simulink model "algorithm"  (R2026a)
settings: Solver=FixedStepDiscrete  FixedStep=foc.Ts
PreLoadFcn:
  | if exist('init', 'file') ~= 2,   pDir = fileparts(fileparts(which(bdroot)));   if isempty(pDir), pDir = pwd; end;   addpath(fullfile(pDir, 'scripts'));   addpath(fullfile(pDir, 'models'));   addpath(pDir); end; init;
InitFcn:
  | if exist('init', 'file') ~= 2,   pDir = fileparts(fileparts(which(bdroot)));   if isempty(pDir), pDir = pwd; end;   addpath(fullfile(pDir, 'scripts'));   addpath(fullfile(pDir, 'models'));   addpath(pDir); end; init;
undefined symbols (not defined in the file): calibration_modulation, calibration_request, control_enable_request, control_fault_reset, control_mode_request, current_offset_counts, DiscIntNeverNeededParam, foc, has_stored_resolver_offset, open_loop_electrical_hz, open_loop_modulation, pmsm, resolver_angle_offset, sensor, torque_ref_nm
libraries: mcbeeMathTransformLib x3, slpidlib x3, mcbcontrolslib x3, simulink x2, mcbpositiondecoderlib x1
(part 1 of 2)
settings Model: Creator=niklasprobst  LastModifiedBy=probst
settings OptimizationCC: DefaultUnderspecifiedDataType=single
settings DebuggingCC: ParameterDowncastMsg=none  ParameterPrecisionLossMsg=none  BusObjectLabelMismatch=error
settings RTWCC: SystemTargetFile=ert.tlc  GenCodeOnly=on  Description=Embedded Coder
settings ERTTargetCC: SupportAbsoluteTime=off  SupportNonFinite=off

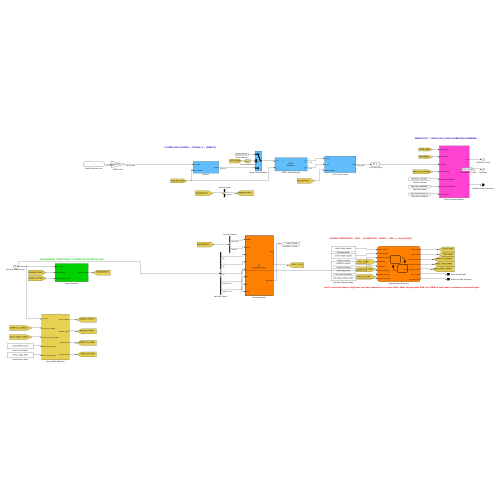
[thumbnail: Simulink's stored preview of the top-level diagram]
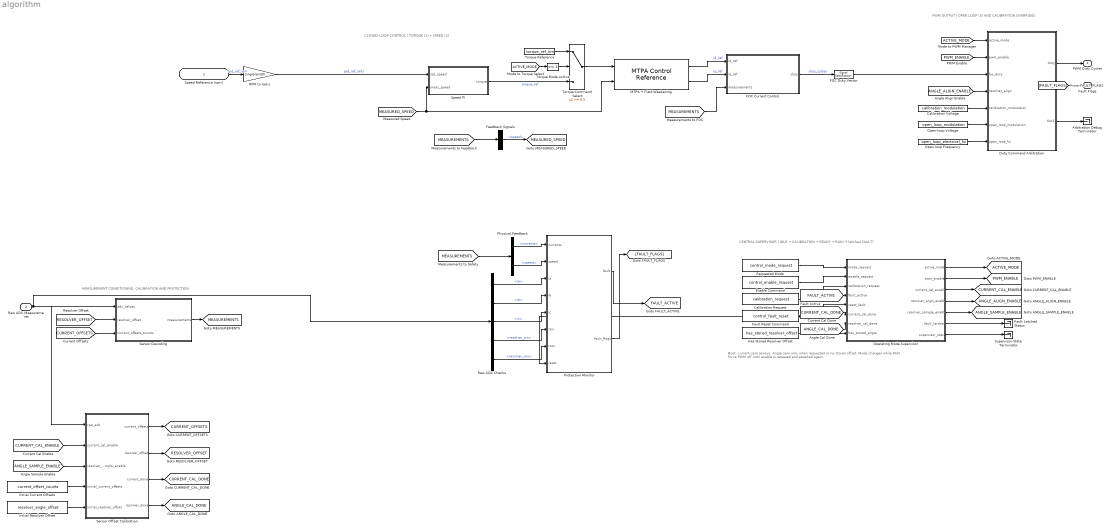
== system algorithm ==
  note: CLOSED-LOOP CONTROL | TORQUE (1) • SPEED (2)
  note: PWM OUTPUT | OPEN LOOP (3) AND CALIBRATION OVERRIDES
  note: MEASUREMENT CONDITIONING, CALIBRATION AND PROTECTION
  note: CENTRAL SUPERVISOR | IDLE → CALIBRATION → READY → RUN (+ latched FAULT)
  note: Boot: current-zero always. Angle-zero only when requested or no stored offset. Mode changes while RUN force PWM off until enable is released and asserted again.
  Speed Reference (rpm) : Inport  OutDataTypeStr=single
  Raw ADC Measurements : Inport  Port=2  OutDataTypeStr=Bus: adc_values
  Arbitration Debug Terminator : Terminator
      settings: Tag=algorithm_clean_routing
  Calibration Request : Constant  Value=calibration_request  OutDataTypeStr=uint8
  Calibration Voltage : Constant  Value=calibration_modulation  OutDataTypeStr=single
  Duty Command Arbitration : Subsystem
  Enable Command : Constant  Value=control_enable_request  OutDataTypeStr=boolean
  FOC Current Control : Subsystem
  FOC Duty Vector : SignalSpecification  Dimensions=3
  Fault Latched Status : Terminator
  Fault Reset Command : Constant  Value=control_fault_reset  OutDataTypeStr=boolean
  Feedback Signals : BusSelector  OutputSignals=speed
  Has Stored Resolver Offset : Constant  Value=has_stored_resolver_offset  OutDataTypeStr=boolean
  Initial Current Offsets : Constant  Value=current_offset_counts  OutDataTypeStr=single
  Initial Resolver Offset : Constant  Value=resolver_angle_offset  OutDataTypeStr=single
  MTPA + Field Weakening : mcbcontrolslib/MTPA Control Reference  VariantSelect=Interior PMSM  polePairs=pmsm.P  Rs=pmsm.Rs  Ld=pmsm.Ld  Lq=pmsm.Lq  FluxPM=pmsm.fl  ilimit=pmsm.I_rated  Vdc_input_select=Specify via dialog  V_dc=pmsm.V_rated  Units=SI Units  N_base=pmsm.N_base  I_base=pmsm.I_rated  T_base=1  V_base=pmsm.V_rated/sqrt(3)  N_base_disp=pmsm.N_base  MTPAiterator=on  iterCount=10
  Open-loop Frequency : Constant  Value=open_loop_electrical_hz  OutDataTypeStr=single
  Open-loop Voltage : Constant  Value=open_loop_modulation  OutDataTypeStr=single
  Operating Mode Supervisor : Stateflow chart  TreatAsAtomicUnit=on
  Physical Feedback : BusSelector  OutputSignals=currents,speed
  Protection Monitor : MATLAB Function  TreatAsAtomicUnit=on
  RPM to rad-s : Gain  Gain=single(pi/30)  OutDataTypeStr=single
  Raw ADC Checks : BusSelector  OutputSignals=ia,ib,ic,resolver_sin,resolver_cos
  Requested Mode : Constant  Value=control_mode_request  OutDataTypeStr=uint8
  Sensor Decoding : Subsystem  Description=|
      | EVADC TO PHYSICAL SENSOR MEASUREMENT CONDITIONING
      | =================================================
      | 1. WHAT IT DOES:
      | Hardware abstraction interface that transforms raw 12-bit integer counts from the
      | Infineon AURIX TC387 EVADC into single-precision physical SI measurements packed into
      | the 'algo_measurement' bus.
      | 
      | 2. INTERFACE SIGNALS:
      | - Input:  'adc_values' bus (uint16 channels: ia, ib, ic, resolver_sin, resolver_cos)
      | - Output: 'measurements' bus (algo_measurement):
      |     * currents [A]    : 3-phase stator currents (Phase A, B, C)
      |     * MtrPos   [rad]  : Mechanical rotor angle in [0, 2*pi)
      |     * speed    [rad/s]: Filtered mechanical rotor speed
      | 
      | 3. INTERNAL SUBMODULES:
      |   1) Current measurement: Signed offset removal & scaling (0..4095 counts -> -120..+120 A).
      |   2) Position measurement: Center removal, normalization, atan2, and [0, 2*pi) wrapping.
      |   3) Speed from position: Differentiator with circular 2*pi unwrapping & 150 Hz LPF.
      | 
      | 4. WHY IT IS NEEDED:
      | Decouples microcontroller register hardware formats from core FOC algorithms, ensuring
      | pure single-precision floating-point execution, determinism, and seamless code generation.
      | Execution rate: Ts = 50 us (20 kHz).
  Sensor Offset Calibration : Subsystem
  Speed PI : Subsystem
  Supervisor State Terminator : Terminator
  Torque Command Select : Switch  Threshold=0.5  SaturateOnIntegerOverflow=off  InputSameDT=off
  Torque Mode Active : simulink/Logic and Bit Operations/Compare To Constant  relop===  const=1  OutDataTypeStr=boolean
  Torque Reference : Constant  Value=torque_ref_nm  OutDataTypeStr=single
  PWM Duty Cycles : Outport  OutDataTypeStr=single
  Fault Flags : Outport  Port=2  OutDataTypeStr=uint32
  tag scope: ACTIVE_MODE=global, ANGLE_ALIGN_ENABLE=global, ANGLE_CAL_DONE=global, ANGLE_SAMPLE_ENABLE=global, CURRENT_CAL_DONE=global, CURRENT_CAL_ENABLE=global, CURRENT_OFFSETS=global, FAULT_ACTIVE=global, MEASURED_SPEED=global, MEASUREMENTS=global, PWM_ENABLE=global, RESOLVER_OFFSET=global
  wires:
  Speed Reference (rpm)/1 -> RPM to rad-s/1  "spd_ref_rpm"
  RPM to rad-s/1 -> Speed PI/1(set_speed)  "spd_ref_rads"
  [MEASURED_SPEED] -> Speed PI/2(meas_speed), MTPA + Field Weakening/2
  Torque Reference/1 -> Torque Command Select/1
  [ACTIVE_MODE] -> Torque Mode Active/1
  Torque Mode Active/1 -> Torque Command Select/2
  Speed PI/1(torque) -> Torque Command Select/3  "torque_ref"
  Torque Command Select/1 -> MTPA + Field Weakening/1
  MTPA + Field Weakening/1 -> FOC Current Control/1(id_ref)  "id_ref"
  MTPA + Field Weakening/2 -> FOC Current Control/2(iq_ref)  "iq_ref"
  [MEASUREMENTS] -> FOC Current Control/3(measurements)
  FOC Current Control/1(duty) -> FOC Duty Vector/1  "duty_cycles"
  FOC Duty Vector/1 -> Duty Command Arbitration/3(foc_duty)
  [ACTIVE_MODE] -> Duty Command Arbitration/1(active_mode)
  [PWM_ENABLE] -> Duty Command Arbitration/2(pwm_enable)
  [ANGLE_ALIGN_ENABLE] -> Duty Command Arbitration/4(resolver_align)
  Calibration Voltage/1 -> Duty Command Arbitration/5(calibration_modulation)
  Open-loop Voltage/1 -> Duty Command Arbitration/6(open_loop_modulation)
  Open-loop Frequency/1 -> Duty Command Arbitration/7(open_loop_hz)
  Duty Command Arbitration/1(duty) -> PWM Duty Cycles/1
  Duty Command Arbitration/2(Out1) -> Arbitration Debug Terminator/1
  Sensor Decoding/1(measurements) -> [MEASUREMENTS]
  [RESOLVER_OFFSET] -> Sensor Decoding/2(resolver_offset)
  [CURRENT_OFFSETS] -> Sensor Decoding/3(current_offsets_counts)
  [MEASUREMENTS] -> Feedback Signals/1
  Feedback Signals/1 -> [MEASURED_SPEED]  "<speed>"
  [MEASUREMENTS] -> Physical Feedback/1
  Physical Feedback/1 -> Protection Monitor/1(currents)  "<currents>"
  Physical Feedback/2 -> Protection Monitor/2(speed)  "<speed>"
  Raw ADC Checks/1 -> Protection Monitor/3(ia)  "<ia>"
  Raw ADC Checks/2 -> Protection Monitor/4(ib)  "<ib>"
  Raw ADC Checks/3 -> Protection Monitor/5(ic)  "<ic>"
  Raw ADC Checks/4 -> Protection Monitor/6(rsin)  "<resolver_sin>"
  Raw ADC Checks/5 -> Protection Monitor/7(rcos)  "<resolver_cos>"
  Protection Monitor/1(fault) -> [FAULT_ACTIVE]
  [CURRENT_CAL_ENABLE] -> Sensor Offset Calibration/2(current_cal_enable)
  [ANGLE_SAMPLE_ENABLE] -> Sensor Offset Calibration/3(resolver_sample_enable)
  Initial Current Offsets/1 -> Sensor Offset Calibration/4(initial_current_offsets)
  Initial Resolver Offset/1 -> Sensor Offset Calibration/5(initial_resolver_offset)
  Sensor Offset Calibration/1(current_offsets) -> [CURRENT_OFFSETS]
  Sensor Offset Calibration/2(resolver_offset) -> [RESOLVER_OFFSET]
  Sensor Offset Calibration/3(current_done) -> [CURRENT_CAL_DONE]
  Sensor Offset Calibration/4(resolver_done) -> [ANGLE_CAL_DONE]
  Requested Mode/1 -> Operating Mode Supervisor/1(mode_request)
  Enable Command/1 -> Operating Mode Supervisor/2(enable_request)
  Calibration Request/1 -> Operating Mode Supervisor/3(calibration_request)
  [FAULT_ACTIVE] -> Operating Mode Supervisor/4(fault_active)
  Fault Reset Command/1 -> Operating Mode Supervisor/5(reset_fault), Protection Monitor/8(reset)
  [CURRENT_CAL_DONE] -> Operating Mode Supervisor/6(current_cal_done)
  [ANGLE_CAL_DONE] -> Operating Mode Supervisor/7(resolver_cal_done)
  Has Stored Resolver Offset/1 -> Operating Mode Supervisor/8(has_stored_angle)
  Operating Mode Supervisor/1(active_mode) -> [ACTIVE_MODE]
  Operating Mode Supervisor/2(pwm_enable) -> [PWM_ENABLE]
  Operating Mode Supervisor/3(current_cal_enable) -> [CURRENT_CAL_ENABLE]
  Operating Mode Supervisor/4(resolver_align_enable) -> [ANGLE_ALIGN_ENABLE]
  Operating Mode Supervisor/5(resolver_sample_enable) -> [ANGLE_SAMPLE_ENABLE]
  Operating Mode Supervisor/6(fault_latched) -> Fault Latched Status/1
  Operating Mode Supervisor/7(supervisor_state) -> Supervisor State Terminator/1
  Raw ADC Measurements/1 -> Sensor Decoding/1(adc_values), Sensor Offset Calibration/1(raw_adc), Raw ADC Checks/1
  Protection Monitor/2(fault_flags) -> [FAULT_FLAGS]
  [FAULT_FLAGS] -> Fault Flags/1

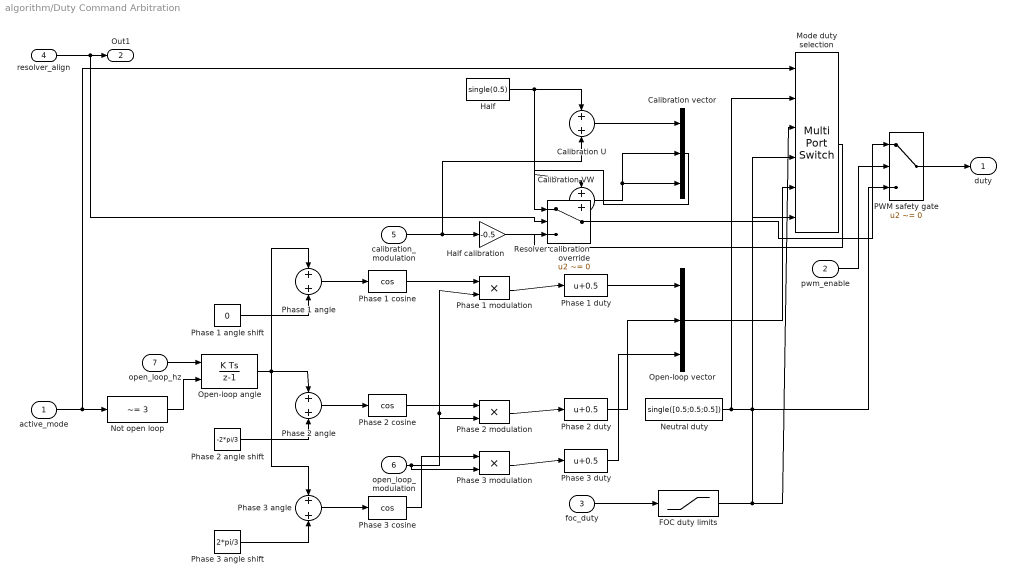
== system algorithm/Duty Command Arbitration ==
  active_mode : Inport
  pwm_enable : Inport  Port=2
  foc_duty : Inport  Port=3
  resolver_align : Inport  Port=4
  calibration_modulation : Inport  Port=5
  open_loop_modulation : Inport  Port=6
  open_loop_hz : Inport  Port=7
  Calibration U : Sum
  Calibration VW : Sum
  Calibration vector : Mux  Inputs=3
  FOC duty limits : Saturate  UpperLimit=0.98  LowerLimit=0.02
  Half : Constant  Value=single(0.5)
  Half calibration : Gain  Gain=-0.5
  Mode duty selection : MultiPortSwitch  DataPortOrder=Zero-based contiguous  Inputs=5  zeroidx=on  SaturateOnIntegerOverflow=off  InputSameDT=off
  Neutral duty : Constant  Value=single([0.5;0.5;0.5])
  Not open loop : simulink/Logic and Bit Operations/Compare To Constant  relop=~=  const=3  OutDataTypeStr=boolean
  Open-loop angle : DiscreteIntegrator  gainval=2*pi  ExternalReset=rising  SampleTime=foc.Ts  LimitOutput=on  UpperSaturationLimit=2*pi  LowerSaturationLimit=0  ICPrevOutput=DiscIntNeverNeededParam  ICPrevScaledInput=DiscIntNeverNeededParam
  Open-loop vector : Mux  Inputs=3
  PWM safety gate : Switch  Criteria=u2 ~= 0  Threshold=0.5  SaturateOnIntegerOverflow=off  InputSameDT=off
  Phase 1 angle : Sum
  Phase 1 angle shift : Constant  Value=0
  Phase 1 cosine : Trigonometry  Operator=cos
  Phase 1 duty : Bias  Bias=0.5  SaturateOnIntegerOverflow=off
  Phase 1 modulation : Product
  Phase 2 angle : Sum
  Phase 2 angle shift : Constant  Value=-2*pi/3
  Phase 2 cosine : Trigonometry  Operator=cos
  Phase 2 duty : Bias  Bias=0.5  SaturateOnIntegerOverflow=off
  Phase 2 modulation : Product
  Phase 3 angle : Sum
  Phase 3 angle shift : Constant  Value=2*pi/3
  Phase 3 cosine : Trigonometry  Operator=cos
  Phase 3 duty : Bias  Bias=0.5  SaturateOnIntegerOverflow=off
  Phase 3 modulation : Product
  Resolver calibration override : Switch  Criteria=u2 ~= 0  SaturateOnIntegerOverflow=off  InputSameDT=off
  duty : Outport
  Out1 : Outport  Port=2
  wires:
  PWM safety gate/1 -> duty/1
  pwm_enable/1 -> PWM safety gate/2
  Neutral duty/1 -> PWM safety gate/3, Mode duty selection/6, Mode duty selection/2
  foc_duty/1 -> FOC duty limits/1
  Phase 3 duty/1 -> Open-loop vector/3
  Phase 2 duty/1 -> Open-loop vector/2
  Phase 1 duty/1 -> Open-loop vector/1
  Half/1 -> Calibration U/1, Calibration VW/1
  Calibration U/1 -> Calibration vector/1
  Calibration VW/1 -> Calibration vector/3, Calibration vector/2
  Phase 3 cosine/1 -> Phase 3 modulation/1
  Phase 3 modulation/1 -> Phase 3 duty/1
  open_loop_modulation/1 -> Phase 2 modulation/2, Phase 1 modulation/2, Phase 3 modulation/2
  Half calibration/1 -> Calibration VW/2
  Phase 2 cosine/1 -> Phase 2 modulation/1
  Phase 1 cosine/1 -> Phase 1 modulation/1
  Phase 1 modulation/1 -> Phase 1 duty/1
  calibration_modulation/1 -> Half calibration/1, Calibration U/2
  Phase 2 modulation/1 -> Phase 2 duty/1
  Phase 3 angle/1 -> Phase 3 cosine/1
  Phase 3 angle shift/1 -> Phase 3 angle/2
  Open-loop angle/1 -> Phase 3 angle/1, Phase 1 angle/1, Phase 2 angle/1
  Phase 1 angle shift/1 -> Phase 1 angle/2
  Not open loop/1 -> Open-loop angle/2
  Phase 1 angle/1 -> Phase 1 cosine/1
  open_loop_hz/1 -> Open-loop angle/1
  active_mode/1 -> Not open loop/1, Mode duty selection/1
  resolver_align/1 -> Out1/1, Resolver calibration override/2
  Phase 2 angle shift/1 -> Phase 2 angle/2
  Phase 2 angle/1 -> Phase 2 cosine/1
  FOC duty limits/1 -> Mode duty selection/3, Mode duty selection/4
  Open-loop vector/1 -> Mode duty selection/5
  Calibration vector/1 -> Resolver calibration override/1
  Mode duty selection/1 -> Resolver calibration override/3
  Resolver calibration override/1 -> PWM safety gate/1

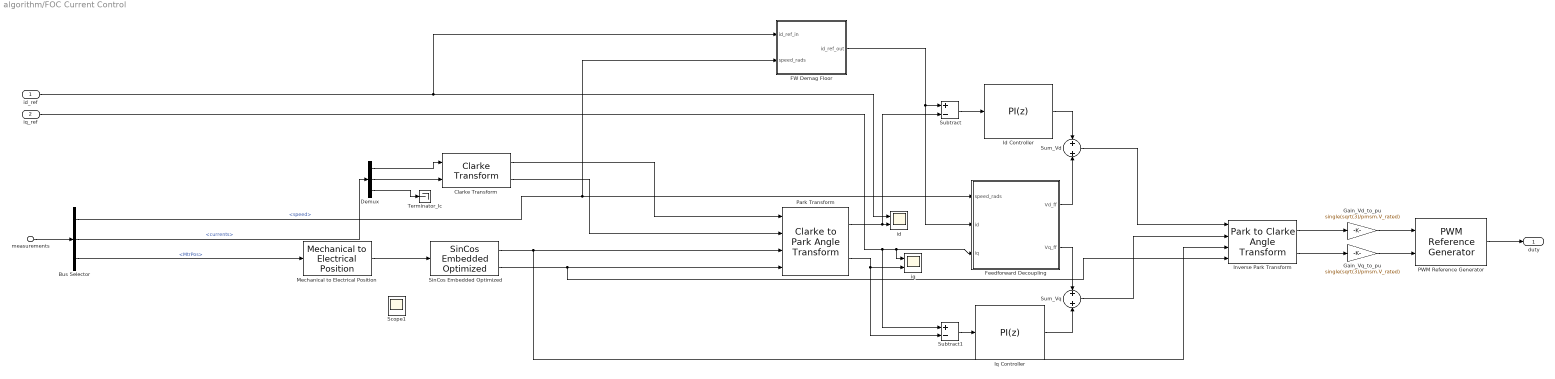
== system algorithm/FOC Current Control ==
  id_ref : Inport
  iq_ref : Inport  Port=2
  measurements : Inport  Port=3  OutDataTypeStr=Bus: algo_measurement
  Bus Selector : BusSelector  OutputSignals=speed,currents,MtrPos
  Clarke Transform : mcbeeMathTransformLib/Clarke Transform  VariantControl=Variant2  PowerInvariant=off  UseWithEmbedded=on  PhaseInput=Two inputs
      settings: LibrarySourceBlock=mcblib/Controls/Math Transforms/Clarke Transform
  Demux : Demux  Outputs=[1 1 1]
  FW Demag Floor : Subsystem  Description=|
      | FIELD WEAKENING DEMAGNETIZATION FLOOR (PHYSICAL VOLTAGE ENVELOPE)
      | =================================================================
      | 1. WHAT IT DOES:
      | Computes the maximum permissible stator flux linkage for the current rotor speed
      | given the inverter voltage headroom, calculates the minimum negative d-axis
      | demagnetization current required to stay within that flux limit, and enforces this
      | floor on id_ref.
      | 
      | 2. MATHEMATICAL FORMULAS:
      |   omega_e      = P * |omega_m|
      |   omega_e_safe = max(omega_e, 100 rad/s)          [Zero-speed division guard]
      |   V_max        = V_phase_max = 0.92 * V_dc / sqrt(3) ≈ 318.7 V
      | 
      | Maximum allowable stator flux linkage before voltage saturation:
      |   lambda_max   = V_max / omega_e_safe
      | 
      | Required d-axis current to suppress stator flux to lambda_max:
      |   i_d_floor_raw = (lambda_max - lambda_pm) / L_d
      |   i_d_floor     = min(0, i_d_floor_raw)           [No positive FW magnetizing current]
      | 
      | Effective d-axis current reference output:
      |   id_ref_out   = min(id_ref_in, i_d_floor)        [Enforces minimum negative d-axis floor]
      | 
      | 3. WHY IT IS NEEDED:
      | - Open-Circuit Back-EMF Overvoltage: Above base speed (N_base ≈ 9,500 RPM), the rotor
      |   PM flux generates a back-EMF (omega_e * lambda_pm) exceeding available phase voltage.
      |   At 18,000-20,000 RPM, back-EMF exceeds 450-500 V against a 318.7 V inverter limit.
      | - Inverter Saturation Prevention: If the speed/MTPA loop cannot request negative i_d
      |   fast enough during rapid acceleration, the inverter saturates, current regulation
      |   collapses, and catastrophic uncontrolled braking/regeneration occurs.
      | - Deterministic Safety Floor: FW Demag Floor acts as an instantaneous, feedforward
      |   physical constraint that guarantees stator terminal back-EMF remains feasible at all RPM.
  Feedforward Decoupling : Subsystem  Description=|
      | FIELD-ORIENTED CONTROL: FEEDFORWARD VOLTAGE DECOUPLING
      | ======================================================
      | 1. WHAT IT DOES:
      | Computes and injects speed-dependent cross-coupling and rotor back-EMF feedforward
      | voltages (Vd_ff, Vq_ff) directly into the d- and q-axis voltage commands.
      | 
      | 2. GOVERNING MOTOR EQUATIONS (Synchronous Rotor dq-Frame):
      |   v_d = R_s * i_d + L_d * (di_d/dt) - omega_e * L_q * i_q
      |   v_q = R_s * i_q + L_q * (di_q/dt) + omega_e * L_d * i_d + omega_e * lambda_pm
      | 
      | where:
      |   omega_e   = P * omega_m         [Electrical angular speed, rad/s]
      |   P         = 4                   [Pole pairs]
      |   L_d, L_q  = 0.35 mH, 0.55 mH    [Direct and quadrature axis inductances]
      |   lambda_pm = 0.0604 Wb           [Permanent magnet flux linkage]
      | 
      | 3. FEEDFORWARD DECOUPLING FORMULAS:
      |   Vd_ff = - omega_e * L_q * i_q
      |   Vq_ff = + omega_e * (L_d * i_d + lambda_pm)
      | 
      | Voltage commands to inverter:
      |   v_d* = v_d_PI + Vd_ff
      |   v_q* = v_q_PI + Vq_ff
      | 
      | 4. WHY IT IS NEEDED:
      | - Nonlinear Decoupling: In IPMSMs, d and q dynamics are strongly coupled through
      |   rotor velocity. Without feedforward, i_q transients disturb i_d and vice versa.
      | - High-Speed Back-EMF & Cross-Coupling Rejection: At maximum speed (20,000 RPM),
      |   omega_e reaches ~8,377 rad/s, producing back-EMF > 500 V and cross-coupling > 200 V.
      |   Without feedforward, the feedback PI integrators must synthesize these huge voltages
      |   purely through tracking error, resulting in severe phase lag, overshoot, and windup.
      | - Ideal Linear SISO Plant: Feedforward cancels the coupling voltages, reducing the
      |   plant seen by the PI controllers to two independent linear first-order SISO loops:
      |     v_d_PI ≈ R_s * i_d + L_d * (di_d/dt)
      |     v_q_PI ≈ R_s * i_q + L_q * (di_q/dt)
      |   ensuring uniform 800 Hz current loop bandwidth across the entire speed envelope.
  Gain_Vd_to_pu : Gain  Gain=single(sqrt(3)/pmsm.V_rated)  OutDataTypeStr=single
  Gain_Vq_to_pu : Gain  Gain=single(sqrt(3)/pmsm.V_rated)  OutDataTypeStr=single
  Id Controller : slpidlib/PID Controller  Controller=PI  Form=Parallel  TimeDomain=Discrete-time  UseExternalTs=off  SampleTime=foc.Ts  IntegratorMethod=Forward Euler  FilterMethod=Forward Euler  ControllerParametersSource=internal  P=foc.Kp_d  I=foc.Ki_d_Ts  UseKiTs=on  D=0  UseExternalDerivativeSource=off  N=100  UseFilter=on  TunerSelectOption=Transfer Function Based (PID Tuner App)  InitialConditionSource=internal  InitialConditionForIntegrator=0  InitialConditionForFilter=0  DifferentiatorICPrevScaledInput=0  ExternalReset=none  TrackingMode=off  Kt=1  LimitOutput=on  SatLimitsSource=internal  UpperSaturationLimit=foc.V_phase_max  LowerSaturationLimit=-foc.V_phase_max  LinearizeAsGain=on  AntiWindupMode=clamping  Kb=0.56841  LimitIntegrator=on  UpperIntegratorSaturationLimit=foc.V_phase_max  LowerIntegratorSaturationLimit=-foc.V_phase_max  RndMeth=Simplest  POutMin=[]  POutMax=[]  IOutMin=[]  IOutMax=[]  DOutMin=[]  DOutMax=[]  NOutMin=[]  NOutMax=[]  SumOutMin=[]  SumOutMax=[]  SaturationOutDataTypeStr=Inherit: Inherit via back propagation  SaturationOutMin=[]  SaturationOutMax=[]  PParamMin=[]  PParamMax=[]  IParamMin=[]  IParamMax=[]  DParamMin=[]  DParamMax=[]  NParamMin=[]  NParamMax=[]  KbParamMin=[]  KbParamMax=[]  KtParamMin=[]  KtParamMax=[]  KbOutMin=[]  KbOutMax=[]  KtOutMin=[]  KtOutMax=[]  IntegratorOutMin=[]  IntegratorOutMax=[]  FilterOutMin=[]  FilterOutMax=[]  SumI1OutMin=[]  SumI1OutMax=[]  SumI2OutMin=[]  SumI2OutMax=[]  SumI3OutMin=[]  SumI3OutMax=[]  SumI4OutMin=[]  SumI4OutMax=[]  SumDOutMin=[]  SumDOutMax=[]  DifferentiatorOutMin=[]  DifferentiatorOutMax=[]  FilterDiffOutCoefMin=[]  FilterDiffOutCoefMax=[]  ReciprocalOutMin=[]  ReciprocalOutMax=[]  SumDenOutMin=[]  SumDenOutMax=[]  SumNumOutMin=[]  SumNumOutMax=[]  DivideOutMin=[]  DivideOutMax=[]  UdiffTsProdOutMin=[]  UdiffTsProdOutMax=[]  NTsProdOutMin=[]  NTsProdOutMax=[]  UintegralTsProdOutMin=[]  UintegralTsProdOutMax=[]  UngainTsProdOutMin=[]  UngainTsProdOutMax=[]  ClampingZeroOutDataTypeStr=Inherit: Inherit via back propagation  ClampingZeroOutMin=[]  ClampingZeroOutMax=[]  FilterDenConstantOutDataTypeStr=Inherit: Inherit via back propagation  FilterDenConstantOutMin=[]  FilterDenConstantOutMax=[]  PCopyOutDataTypeStr=Inherit: Inherit via back propagation  PCopyOutMin=[]  PCopyOutMax=[]  NCopyOutDataTypeStr=Inherit: Inherit via back propagation  NCopyOutMin=[]  NCopyOutMax=[]  IntegratorContinuousStateAttributes=''  IntegratorStateMustResolveToSignalObject=off  IntegratorRTWStateStorageClass=Auto  FilterContinuousStateAttributes=''  FilterStateMustResolveToSignalObject=off  FilterRTWStateStorageClass=Auto  ParallelPVariant=InternalParameters  IdealPVariant=Disabled  IVariant=InternalParameters  DVariant=Disabled  IntegratorVariant=Discrete  SatVariant=Enabled  AWVariant=DiscClampingParallel  PCopyVariant=Disabled  TRVariant=Disabled  FdbkBlocksVariant=Forward  IdealPFdbkVariant=Disabled  SatFdbkVariant=Disabled  DerivativeFilterVariant=Disabled  NVariant=Disabled  NCopyVariant=Disabled_SignalSpec  FilterICVariant=Disabled  IntegratorICVariant=InternalICs  ExternalResetVariant=Disabled  TRSumVariant=Passthrough  SumFdbkVariant=Disabled  SumVariant=Sum_PI  TsampFilterVariant=InternalTs  TsampNgainVariant=Passthrough  TsampIntegralVariant=Disabled_SignalSpec  ExternalSaturationOutDataTypeStr=Inherit: Same as second input  DerivativeSourceVariant=Disabled  PreIntVariant=InternalPreInt
      settings: LibrarySourceBlock=mcblib/Controls/Controllers/PI Controller
  Inverse Park Transform : mcbeeMathTransformLib/Park to Clarke Angle Transform  AxisAlignment=D-axis  UseWithEmbedded=on  PhaseInput=Two inputs  ThetaInput=Sine and Cosine electrical position  AngleInput=Per-unit  N_points=1024
      settings: LibrarySourceBlock=mcblib/Controls/Math Transforms/Inverse Park Transform
  Iq Controller : slpidlib/PID Controller  Controller=PI  Form=Parallel  TimeDomain=Discrete-time  UseExternalTs=off  SampleTime=foc.Ts  IntegratorMethod=Forward Euler  FilterMethod=Forward Euler  ControllerParametersSource=internal  P=foc.Kp_q  I=foc.Ki_q_Ts  UseKiTs=on  D=0  UseExternalDerivativeSource=off  N=100  UseFilter=on  TunerSelectOption=Transfer Function Based (PID Tuner App)  InitialConditionSource=internal  InitialConditionForIntegrator=0  InitialConditionForFilter=0  DifferentiatorICPrevScaledInput=0  ExternalReset=none  TrackingMode=off  Kt=1  LimitOutput=on  SatLimitsSource=internal  UpperSaturationLimit=foc.V_phase_max  LowerSaturationLimit=-foc.V_phase_max  LinearizeAsGain=on  AntiWindupMode=clamping  Kb=0.36172  LimitIntegrator=on  UpperIntegratorSaturationLimit=foc.V_phase_max  LowerIntegratorSaturationLimit=-foc.V_phase_max  RndMeth=Simplest  POutMin=[]  POutMax=[]  IOutMin=[]  IOutMax=[]  DOutMin=[]  DOutMax=[]  NOutMin=[]  NOutMax=[]  SumOutMin=[]  SumOutMax=[]  SaturationOutDataTypeStr=Inherit: Inherit via back propagation  SaturationOutMin=[]  SaturationOutMax=[]  PParamMin=[]  PParamMax=[]  IParamMin=[]  IParamMax=[]  DParamMin=[]  DParamMax=[]  NParamMin=[]  NParamMax=[]  KbParamMin=[]  KbParamMax=[]  KtParamMin=[]  KtParamMax=[]  KbOutMin=[]  KbOutMax=[]  KtOutMin=[]  KtOutMax=[]  IntegratorOutMin=[]  IntegratorOutMax=[]  FilterOutMin=[]  FilterOutMax=[]  SumI1OutMin=[]  SumI1OutMax=[]  SumI2OutMin=[]  SumI2OutMax=[]  SumI3OutMin=[]  SumI3OutMax=[]  SumI4OutMin=[]  SumI4OutMax=[]  SumDOutMin=[]  SumDOutMax=[]  DifferentiatorOutMin=[]  DifferentiatorOutMax=[]  FilterDiffOutCoefMin=[]  FilterDiffOutCoefMax=[]  ReciprocalOutMin=[]  ReciprocalOutMax=[]  SumDenOutMin=[]  SumDenOutMax=[]  SumNumOutMin=[]  SumNumOutMax=[]  DivideOutMin=[]  DivideOutMax=[]  UdiffTsProdOutMin=[]  UdiffTsProdOutMax=[]  NTsProdOutMin=[]  NTsProdOutMax=[]  UintegralTsProdOutMin=[]  UintegralTsProdOutMax=[]  UngainTsProdOutMin=[]  UngainTsProdOutMax=[]  ClampingZeroOutDataTypeStr=Inherit: Inherit via back propagation  ClampingZeroOutMin=[]  ClampingZeroOutMax=[]  FilterDenConstantOutDataTypeStr=Inherit: Inherit via back propagation  FilterDenConstantOutMin=[]  FilterDenConstantOutMax=[]  PCopyOutDataTypeStr=Inherit: Inherit via back propagation  PCopyOutMin=[]  PCopyOutMax=[]  NCopyOutDataTypeStr=Inherit: Inherit via back propagation  NCopyOutMin=[]  NCopyOutMax=[]  IntegratorContinuousStateAttributes=''  IntegratorStateMustResolveToSignalObject=off  IntegratorRTWStateStorageClass=Auto  FilterContinuousStateAttributes=''  FilterStateMustResolveToSignalObject=off  FilterRTWStateStorageClass=Auto  ParallelPVariant=InternalParameters  IdealPVariant=Disabled  IVariant=InternalParameters  DVariant=Disabled  IntegratorVariant=Discrete  SatVariant=Enabled  AWVariant=DiscClampingParallel  PCopyVariant=Disabled  TRVariant=Disabled  FdbkBlocksVariant=Forward  IdealPFdbkVariant=Disabled  SatFdbkVariant=Disabled  DerivativeFilterVariant=Disabled  NVariant=Disabled  NCopyVariant=Disabled_SignalSpec  FilterICVariant=Disabled  IntegratorICVariant=InternalICs  ExternalResetVariant=Disabled  TRSumVariant=Passthrough  SumFdbkVariant=Disabled  SumVariant=Sum_PI  TsampFilterVariant=InternalTs  TsampNgainVariant=Passthrough  TsampIntegralVariant=Disabled_SignalSpec  ExternalSaturationOutDataTypeStr=Inherit: Same as second input  DerivativeSourceVariant=Disabled  PreIntVariant=InternalPreInt
      settings: LibrarySourceBlock=mcblib/Controls/Controllers/PI Controller
  Mechanical to Electrical Position : mcbpositiondecoderlib/Mechanical to Electrical Position  PolePairsInputType=Specify via dialog  NrPP=pmsm.P  selectedRange=Radians  MechOfstInputType=Specify via dialog  mechOffsetIn=0  maxAngleIn=2*pi  InputDataType=single  VariantSelect=floating-point
      settings: LibrarySourceBlock=mcblib/Sensor Decoders/Mechanical to Electrical Position
  PWM Reference Generator : mcbcontrolslib/PWM Reference Generator  modType=SVM: space vector modulation  inSignal=Valphabeta  expandVoltageInput=on  inputUnits=Per-unit  LimitModulation=off  enableVoltage=off  enableModulationSignal=off  enableDutyCycle=on  expandVoltageOutput=on
      settings: LibrarySourceBlock=mcblib/Controls/Math Transforms/PWM Reference Generator
  Park Transform : mcbeeMathTransformLib/Clarke to Park Angle Transform  AxisAlignment=D-axis  UseWithEmbedded=on  PhaseInput=Two inputs  ThetaInput=Sine and Cosine electrical position  AngleInput=Per-unit  N_points=1024
      settings: LibrarySourceBlock=mcblib/Controls/Math Transforms/Park Transform
  Scope1 : Scope  NumInputPorts=2
      settings: ActiveDisplayYMinimum=-3.5597814582216527  ActiveDisplayYMaximum=6.3570651964002307  DataLoggingVariableName=ScopeData3
  SinCos Embedded Optimized : mcbcontrolslib/SinCos Embedded Optimized  LabelModeActiveChoice=MCB_Sin  OptforProc=off  OptLevelPop=Disabled  ApproximationMethod=None  UserApproxMethod=Lookup  ApproxStatus=None  ThetaDataType=single  CopyThetaDataType=single  InterpMethod=Linear point-slope  NumberOfDataPoints=16  NumberOfIterations=11  RemoveProtectionAgainstOutOfRangeInput=off  TableDataTypeStr=Inherit: Inherit via input  AngleInput=Radians  CopyAngleInput=Radians  N_points=1024  CopyN_points=1024  Datatype=Inherit: Same as input  CopyTableDatatype=Inherit: Same as input  DatatypeInput=Inherit from input  IsPrevStrictOpt=0  IsPrevLUTForced=0
      settings: LibrarySourceBlock=mcblib/Controls/Math Transforms/SinCos Embedded Optimized
  Subtract : Sum  Inputs=+-
  Subtract1 : Sum  Inputs=+-
  Sum_Vd : Sum
  Sum_Vq : Sum
  Terminator_Ic : Terminator
  id : Scope  NumInputPorts=2
      settings: ActiveDisplayYMinimum=-59.918689407408237  ActiveDisplayYMaximum=7.2363061681389791
  iq : Scope  NumInputPorts=2
      settings: ActiveDisplayYMinimum=-43.481506402956065  ActiveDisplayYMaximum=105.58190007147998  DataLoggingVariableName=ScopeData6
  duty : Outport  PortDimensions=3
  wires:
  Subtract1/1 -> Iq Controller/1
  PWM Reference Generator/1 -> duty/1
  FW Demag Floor/1(id_ref_out) -> Feedforward Decoupling/2(id), Subtract/1
  Bus Selector/1 -> Feedforward Decoupling/1(speed_rads), FW Demag Floor/2(speed_rads)  "<speed>"
  SinCos Embedded Optimized/1 -> Park Transform/3, Inverse Park Transform/3
  Bus Selector/3 -> Mechanical to Electrical Position/1  "<MtrPos>"
  Park Transform/2 -> iq/2, Subtract1/2
  measurements/1 -> Bus Selector/1
  Gain_Vd_to_pu/1 -> PWM Reference Generator/1
  Demux/2 -> Clarke Transform/2
  Mechanical to Electrical Position/1 -> SinCos Embedded Optimized/1
  Demux/3 -> Terminator_Ic/1
  Inverse Park Transform/2 -> Gain_Vq_to_pu/1
  Feedforward Decoupling/1(Vd_ff) -> Sum_Vd/2
  Sum_Vq/1 -> Inverse Park Transform/2
  Clarke Transform/1 -> Park Transform/1
  Bus Selector/2 -> Demux/1  "<currents>"
  Sum_Vd/1 -> Inverse Park Transform/1
  Gain_Vq_to_pu/1 -> PWM Reference Generator/2
  Clarke Transform/2 -> Park Transform/2
  Park Transform/1 -> Subtract/2, id/2
  Inverse Park Transform/1 -> Gain_Vd_to_pu/1
  id_ref/1 -> FW Demag Floor/1(id_ref_in), id/1
  Subtract/1 -> Id Controller/1
  SinCos Embedded Optimized/2 -> Park Transform/4, Inverse Park Transform/4
  Id Controller/1 -> Sum_Vd/1
  Demux/1 -> Clarke Transform/1
  iq_ref/1 -> Subtract1/1, iq/1, Feedforward Decoupling/3(iq)
  Feedforward Decoupling/2(Vq_ff) -> Sum_Vq/1
  Iq Controller/1 -> Sum_Vq/2

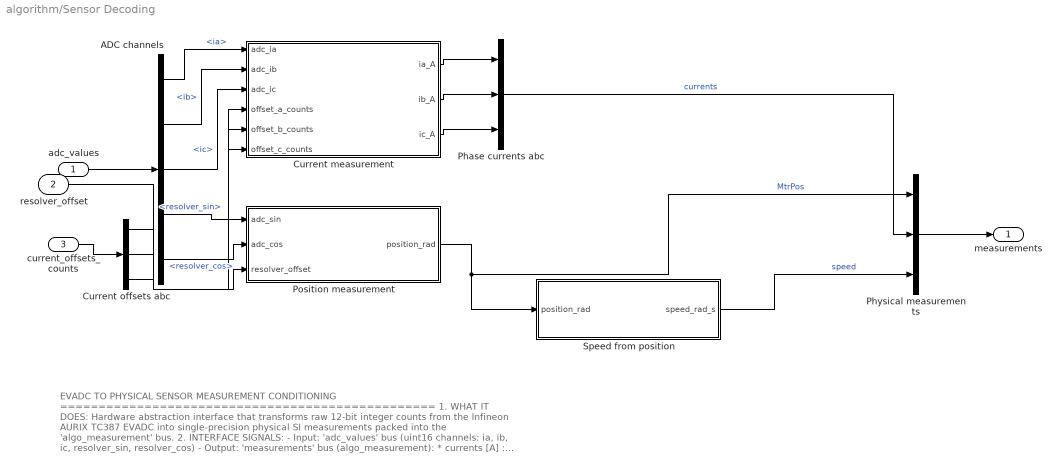
== system algorithm/Sensor Decoding ==
  note: EVADC TO PHYSICAL SENSOR MEASUREMENT CONDITIONING
      | =================================================
      | 1. WHAT IT DOES:
      | Hardware abstraction interface that transforms raw 12-bit integer counts from the
      | Infineon AURIX TC387 EVADC into single-precision physical SI measurements packed into
      | the 'algo_measurement' bus.
      |
      | 2. INTERFACE SIGNALS:
      | - Input:  'adc_values' bus (uint16 channels: ia, ib, ic, resolver_sin, resolver_cos)
      | - Output: 'measurements' bus (algo_measurement):
      |     * currents [A]    : 3-phase stator currents (Phase A, B, C)
      |     * MtrPos   [rad]  : Mechanical rotor angle in [0, 2*pi)
      |     * speed    [rad/s]: Filtered mechanical rotor speed
      |
      | 3. INTERNAL SUBMODULES:
      |   1) Current measurement: Signed offset removal & scaling (0..4095 counts -> -120..+120 A).
      |   2) Position measurement: Center removal, normalization, atan2, and [0, 2*pi) wrapping.
      |   3) Speed from position: Differentiator with circular 2*pi unwrapping & 150 Hz LPF.
      |
      | 4. WHY IT IS NEEDED:
      | Decouples microcontroller register hardware formats from core FOC algorithms, ensuring
      | pure single-precision floating-point execution, determinism, and seamless code generation.
      | Execution rate: Ts = 50 us (20 kHz).
  adc_values : Inport  OutDataTypeStr=Bus: adc_values
  resolver_offset : Inport  Port=2
  current_offsets_counts : Inport  Port=3  PortDimensions=3
  ADC channels : BusSelector  OutputSignals=ia,ib,ic,resolver_sin,resolver_cos
  Current measurement : Subsystem  Description=|
      | STATOR PHASE CURRENT MEASUREMENT & SCALING
      | ==========================================
      | 1. WHAT IT DOES:
      | Converts 12-bit unsigned ADC counts (0..4095) from current sensors into signed
      | phase currents in Amperes for phases A, B, and C.
      | 
      | 2. CONVERSION FORMULA:
      | For each phase k in {a, b, c}:
      |   i_k = (ADC_k - ADC_mid) * (I_max / ADC_span)
      |       = (single(ADC_k) - 2048.0) * (120.0 / 2047.0)  [Amperes]
      | 
      | Calibration parameters (sensor struct):
      |   ADC_mid  = 2048   [Zero-current center code, 2.5 V mid-rail]
      |   ADC_span = 2047   [Unipolar count span]
      |   I_max    = 120.0  [Transducer full-scale current, A]
      | 
      | 3. WHY IT IS NEEDED:
      | Hall-effect current sensors produce an analog voltage centered at 2.5 V (count 2048)
      | for 0 A, swinging between 0 V (count 0, ≈ -120 A) and 5 V (count 4095, +120 A).
      | This block converts discrete integer ADC codes to physical currents for Clarke transformation.
  Current offsets abc : Demux  Outputs=3
  Phase currents abc : Mux  Inputs=3
  Physical measurements : BusCreator  Inputs=3  OutDataTypeStr=Bus: algo_measurement  NonVirtualBus=on
      settings: InheritFromInputs=off
  Position measurement : Subsystem  Description=|
      | RESOLVER ROTOR POSITION DECODING & CIRCULAR WRAPPING
      | ===================================================
      | 1. WHAT IT DOES:
      | Demodulates and converts orthogonal resolver envelope ADC counts into mechanical rotor
      | position angle in radians, strictly wrapped to the single-turn interval [0, 2*pi).
      | 
      | 2. MATHEMATICAL FORMULAS:
      |   sin_norm = (single(adc_sin) - 2048.0) / 2047.0
      |   cos_norm = (single(adc_cos) - 2048.0) / 2047.0
      |   theta_raw = atan2(sin_norm, cos_norm)           [Range: (-pi, +pi] rad]
      |   position_rad = mod(theta_raw, 2*pi)             [Range: [0, 2*pi) rad]
      | 
      | 3. WHY IT IS NEEDED:
      | Field-Oriented Control requires accurate, continuous knowledge of rotor position to align
      | the Park and Clarke reference frames. Using atan2(sin, cos) provides amplitude-invariant
      | angle reconstruction that rejects common-mode excitation variations and noise. Wrapping to
      | [0, 2*pi) provides a clean, standardized mechanical coordinate system for electrical angle derivation.
  Speed from position : Subsystem  Description=|
      | SPEED ESTIMATION: CIRCULAR UNWRAPPING & LOW-PASS FILTERING
      | ==========================================================
      | 1. WHAT IT DOES:
      | Calculates mechanical angular velocity (speed_rad_s) from rotor position samples,
      | unwrapping circular 2*pi phase boundaries, suppressing startup spikes, and filtering
      | quantization noise.
      | 
      | 2. MATHEMATICAL FORMULAS:
      | Sample-to-sample angular difference:
      |   delta_theta = position_rad(k) - position_rad(k-1)
      | 
      | Circular shortest-path unwrapping (handles 0 <-> 2*pi transitions):
      |   delta_theta_unwrap = delta_theta - 2*pi * round(delta_theta / (2*pi))
      | 
      | Differentiated raw speed (with first-step startup suppression):
      |   omega_raw(1) = 0
      |   omega_raw(k) = delta_theta_unwrap / Ts          [Ts = 50 us (20 kHz)]
      | 
      | Discrete 1st-order Low-Pass Filter (cutoff fc = 150 Hz):
      |   omega_filt(k) = (1 - alpha) * omega_filt(k-1) + alpha * omega_raw(k)
      |   alpha = (2*pi * fc * Ts) / (1 + 2*pi * fc * Ts) ≈ 0.04505
      | 
      | 3. WHY IT IS NEEDED:
      | - Boundary Wrap Immunity: As the rotor rotates past 2*pi -> 0 or 0 -> 2*pi, delta_theta
      |   would jump by +/-2*pi, producing an enormous false velocity spike (+/-125,663 rad/s).
      |   Shortest-path unwrapping eliminates this completely.
      | - Startup Quiescence: Suppressing the first step prevents false speed kicks when starting
      |   from a nonzero stationary angle.
      | - Noise Rejection: Differentiating quantized 12-bit ADC resolver signals amplifies high-
      |   frequency quantization noise; the 150 Hz LPF smooths the velocity signal for stable speed
      |   and current loop feedback.
  measurements : Outport  OutDataTypeStr=Bus: algo_measurement
  wires:
  Position measurement/1(position_rad) -> Speed from position/1(position_rad), Physical measurements/1  "MtrPos"
  Current measurement/2(ib_A) -> Phase currents abc/2
  ADC channels/5 -> Position measurement/2(adc_cos)  "<resolver_cos>"
  ADC channels/4 -> Position measurement/1(adc_sin)  "<resolver_sin>"
  adc_values/1 -> ADC channels/1
  ADC channels/3 -> Current measurement/3(adc_ic)  "<ic>"
  Physical measurements/1 -> measurements/1
  Current measurement/1(ia_A) -> Phase currents abc/1
  ADC channels/2 -> Current measurement/2(adc_ib)  "<ib>"
  Current measurement/3(ic_A) -> Phase currents abc/3
  ADC channels/1 -> Current measurement/1(adc_ia)  "<ia>"
  Speed from position/1(speed_rad_s) -> Physical measurements/3  "speed"
  Phase currents abc/1 -> Physical measurements/2  "currents"
  resolver_offset/1 -> Position measurement/3(resolver_offset)
  current_offsets_counts/1 -> Current offsets abc/1
  Current offsets abc/1 -> Current measurement/4(offset_a_counts)
  Current offsets abc/2 -> Current measurement/5(offset_b_counts)
  Current offsets abc/3 -> Current measurement/6(offset_c_counts)

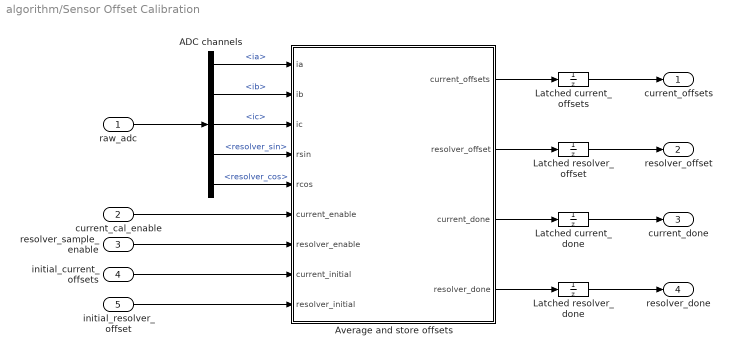
== system algorithm/Sensor Offset Calibration ==
  raw_adc : Inport
  current_cal_enable : Inport  Port=2
  resolver_sample_enable : Inport  Port=3
  initial_current_offsets : Inport  Port=4  PortDimensions=3
  initial_resolver_offset : Inport  Port=5
  ADC channels : BusSelector  OutputSignals=ia,ib,ic,resolver_sin,resolver_cos
  Average and store offsets : MATLAB Function  TreatAsAtomicUnit=on
  Latched current_done : UnitDelay  InitialCondition=false  SampleTime=foc.Ts
  Latched current_offsets : UnitDelay  InitialCondition=current_offset_counts  SampleTime=foc.Ts
  Latched resolver_done : UnitDelay  InitialCondition=false  SampleTime=foc.Ts
  Latched resolver_offset : UnitDelay  InitialCondition=resolver_angle_offset  SampleTime=foc.Ts
  current_offsets : Outport
  resolver_offset : Outport  Port=2
  current_done : Outport  Port=3
  resolver_done : Outport  Port=4
  wires:
  raw_adc/1 -> ADC channels/1
  ADC channels/1 -> Average and store offsets/1(ia)  "<ia>"
  ADC channels/2 -> Average and store offsets/2(ib)  "<ib>"
  ADC channels/3 -> Average and store offsets/3(ic)  "<ic>"
  ADC channels/4 -> Average and store offsets/4(rsin)  "<resolver_sin>"
  ADC channels/5 -> Average and store offsets/5(rcos)  "<resolver_cos>"
  current_cal_enable/1 -> Average and store offsets/6(current_enable)
  resolver_sample_enable/1 -> Average and store offsets/7(resolver_enable)
  initial_current_offsets/1 -> Average and store offsets/8(current_initial)
  initial_resolver_offset/1 -> Average and store offsets/9(resolver_initial)
  Average and store offsets/1(current_offsets) -> Latched current_offsets/1
  Latched current_offsets/1 -> current_offsets/1
  Average and store offsets/2(resolver_offset) -> Latched resolver_offset/1
  Latched resolver_offset/1 -> resolver_offset/1
  Average and store offsets/3(current_done) -> Latched current_done/1
  Latched current_done/1 -> current_done/1
  Average and store offsets/4(resolver_done) -> Latched resolver_done/1
  Latched resolver_done/1 -> resolver_done/1

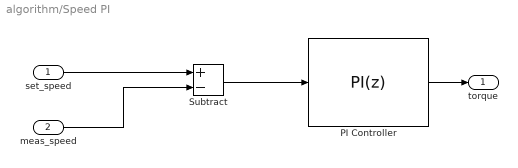
== system algorithm/Speed PI ==
  set_speed : Inport
  meas_speed : Inport  Port=2
  PI Controller : slpidlib/PID Controller  Controller=PI  Form=Parallel  TimeDomain=Discrete-time  UseExternalTs=off  SampleTime=foc.Ts_speed  IntegratorMethod=Forward Euler  FilterMethod=Forward Euler  ControllerParametersSource=internal  P=foc.Kp_spd  I=foc.Ki_spd  UseKiTs=off  D=0  UseExternalDerivativeSource=off  N=100  UseFilter=on  TunerSelectOption=Transfer Function Based (PID Tuner App)  InitialConditionSource=internal  InitialConditionForIntegrator=0  InitialConditionForFilter=0  DifferentiatorICPrevScaledInput=0  ExternalReset=none  TrackingMode=off  Kt=1  LimitOutput=on  SatLimitsSource=internal  UpperSaturationLimit=pmsm.T_peak  LowerSaturationLimit=-pmsm.T_peak  LinearizeAsGain=on  AntiWindupMode=clamping  Kb=10  LimitIntegrator=on  UpperIntegratorSaturationLimit=pmsm.T_peak  LowerIntegratorSaturationLimit=-pmsm.T_peak  RndMeth=Simplest  POutMin=[]  POutMax=[]  IOutMin=[]  IOutMax=[]  DOutMin=[]  DOutMax=[]  NOutMin=[]  NOutMax=[]  SumOutMin=[]  SumOutMax=[]  SaturationOutDataTypeStr=Inherit: Inherit via back propagation  SaturationOutMin=[]  SaturationOutMax=[]  PParamMin=[]  PParamMax=[]  IParamMin=[]  IParamMax=[]  DParamMin=[]  DParamMax=[]  NParamMin=[]  NParamMax=[]  KbParamMin=[]  KbParamMax=[]  KtParamMin=[]  KtParamMax=[]  KbOutMin=[]  KbOutMax=[]  KtOutMin=[]  KtOutMax=[]  IntegratorOutMin=[]  IntegratorOutMax=[]  FilterOutMin=[]  FilterOutMax=[]  SumI1OutMin=[]  SumI1OutMax=[]  SumI2OutMin=[]  SumI2OutMax=[]  SumI3OutMin=[]  SumI3OutMax=[]  SumI4OutMin=[]  SumI4OutMax=[]  SumDOutMin=[]  SumDOutMax=[]  DifferentiatorOutMin=[]  DifferentiatorOutMax=[]  FilterDiffOutCoefMin=[]  FilterDiffOutCoefMax=[]  ReciprocalOutMin=[]  ReciprocalOutMax=[]  SumDenOutMin=[]  SumDenOutMax=[]  SumNumOutMin=[]  SumNumOutMax=[]  DivideOutMin=[]  DivideOutMax=[]  UdiffTsProdOutMin=[]  UdiffTsProdOutMax=[]  NTsProdOutMin=[]  NTsProdOutMax=[]  UintegralTsProdOutMin=[]  UintegralTsProdOutMax=[]  UngainTsProdOutMin=[]  UngainTsProdOutMax=[]  ClampingZeroOutDataTypeStr=Inherit: Inherit via back propagation  ClampingZeroOutMin=[]  ClampingZeroOutMax=[]  FilterDenConstantOutDataTypeStr=Inherit: Inherit via back propagation  FilterDenConstantOutMin=[]  FilterDenConstantOutMax=[]  PCopyOutDataTypeStr=Inherit: Inherit via back propagation  PCopyOutMin=[]  PCopyOutMax=[]  NCopyOutDataTypeStr=Inherit: Inherit via back propagation  NCopyOutMin=[]  NCopyOutMax=[]  IntegratorContinuousStateAttributes=''  IntegratorStateMustResolveToSignalObject=off  IntegratorRTWStateStorageClass=Auto  FilterContinuousStateAttributes=''  FilterStateMustResolveToSignalObject=off  FilterRTWStateStorageClass=Auto  ParallelPVariant=InternalParameters  IdealPVariant=Disabled  IVariant=InternalParameters  DVariant=Disabled  IntegratorVariant=Discrete  SatVariant=Enabled  AWVariant=DiscClampingParallel  PCopyVariant=Disabled  TRVariant=Disabled  FdbkBlocksVariant=Forward  IdealPFdbkVariant=Disabled  SatFdbkVariant=Disabled  DerivativeFilterVariant=Disabled  NVariant=Disabled  NCopyVariant=Disabled_SignalSpec  FilterICVariant=Disabled  IntegratorICVariant=InternalICs  ExternalResetVariant=Disabled  TRSumVariant=Passthrough  SumFdbkVariant=Disabled  SumVariant=Sum_PI  TsampFilterVariant=InternalTs  TsampNgainVariant=Passthrough  TsampIntegralVariant=Disabled_SignalSpec  ExternalSaturationOutDataTypeStr=Inherit: Same as second input  DerivativeSourceVariant=Disabled  PreIntVariant=InternalPreInt
      settings: LibrarySourceBlock=mcblib/Controls/Controllers/PI Controller
  Subtract : Sum  Inputs=+-
  torque : Outport
  wires:
  Subtract/1 -> PI Controller/1
  meas_speed/1 -> Subtract/2
  set_speed/1 -> Subtract/1
  PI Controller/1 -> torque/1

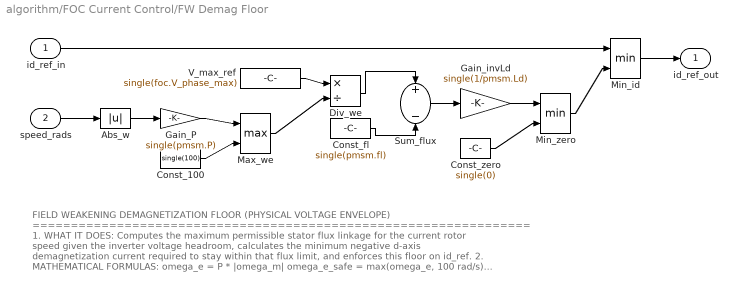
== system algorithm/FOC Current Control/FW Demag Floor ==
  note: FIELD WEAKENING DEMAGNETIZATION FLOOR (PHYSICAL VOLTAGE ENVELOPE)
      | =================================================================
      | 1. WHAT IT DOES:
      | Computes the maximum permissible stator flux linkage for the current rotor speed
      | given the inverter voltage headroom, calculates the minimum negative d-axis
      | demagnetization current required to stay within that flux limit, and enforces this
      | floor on id_ref.
      |
      | 2. MATHEMATICAL FORMULAS:
      |   omega_e      = P * |omega_m|
      |   omega_e_safe = max(omega_e, 100 rad/s)          [Zero-speed division guard]
      |   V_max        = V_phase_max = 0.92 * V_dc / sqrt(3) ≈ 318.7 V
      |
      | Maximum allowable stator flux linkage before voltage saturation:
      |   lambda_max   = V_max / omega_e_safe
      |
      | Required d-axis current to suppress stator flux to lambda_max:
      |   i_d_floor_raw = (lambda_max - lambda_pm) / L_d
      |   i_d_floor     = min(0, i_d_floor_raw)           [No positive FW magnetizing current]
      |
      | Effective d-axis current reference output:
      |   id_ref_out   = min(id_ref_in, i_d_floor)        [Enforces minimum negative d-axis floor]
      |
      | 3. WHY IT IS NEEDED:
      | - Open-Circuit Back-EMF Overvoltage: Above base speed (N_base ≈ 9,500 RPM), the rotor
      |   PM flux generates a back-EMF (omega_e * lambda_pm) exceeding available phase voltage.
      |   At 18,000-20,000 RPM, back-EMF exceeds 450-500 V against a 318.7 V inverter limit.
      | - Inverter Saturation Prevention: If the speed/MTPA loop cannot request negative i_d
      |   fast enough during rapid acceleration, the inverter saturates, current regulation
      |   collapses, and catastrophic uncontrolled braking/regeneration occurs.
      | - Deterministic Safety Floor: FW Demag Floor acts as an instantaneous, feedforward
      |   physical constraint that guarantees stator terminal back-EMF remains feasible at all RPM.
  id_ref_in : Inport
  speed_rads : Inport  Port=2
  Abs_w : Abs  SaturateOnIntegerOverflow=off
  Const_100 : Constant  Value=single(100)  OutDataTypeStr=single
  Const_fl : Constant  Value=single(pmsm.fl)  OutDataTypeStr=single
  Const_zero : Constant  Value=single(0)  OutDataTypeStr=single
  Div_we : Product  Inputs=*/
  Gain_P : Gain  Gain=single(pmsm.P)  OutDataTypeStr=single
  Gain_invLd : Gain  Gain=single(1/pmsm.Ld)  OutDataTypeStr=single
  Max_we : MinMax  Function=max  Inputs=2
  Min_id : MinMax  Inputs=2
  Min_zero : MinMax  Inputs=2
  Sum_flux : Sum  Inputs=+-
  V_max_ref : Constant  Value=single(foc.V_phase_max)  OutDataTypeStr=single
  id_ref_out : Outport
  wires:
  speed_rads/1 -> Abs_w/1
  Abs_w/1 -> Gain_P/1
  Gain_P/1 -> Max_we/1
  Const_100/1 -> Max_we/2
  V_max_ref/1 -> Div_we/1
  Max_we/1 -> Div_we/2
  Div_we/1 -> Sum_flux/1
  Const_fl/1 -> Sum_flux/2
  Sum_flux/1 -> Gain_invLd/1
  Gain_invLd/1 -> Min_zero/1
  Const_zero/1 -> Min_zero/2
  id_ref_in/1 -> Min_id/1
  Min_zero/1 -> Min_id/2
  Min_id/1 -> id_ref_out/1

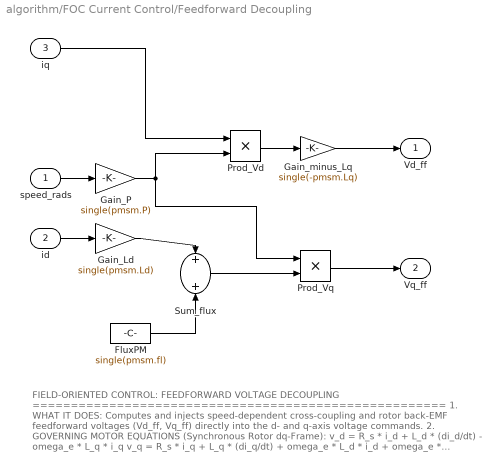
== system algorithm/FOC Current Control/Feedforward Decoupling ==
  note: FIELD-ORIENTED CONTROL: FEEDFORWARD VOLTAGE DECOUPLING
      | ======================================================
      | 1. WHAT IT DOES:
      | Computes and injects speed-dependent cross-coupling and rotor back-EMF feedforward
      | voltages (Vd_ff, Vq_ff) directly into the d- and q-axis voltage commands.
      |
      | 2. GOVERNING MOTOR EQUATIONS (Synchronous Rotor dq-Frame):
      |   v_d = R_s * i_d + L_d * (di_d/dt) - omega_e * L_q * i_q
      |   v_q = R_s * i_q + L_q * (di_q/dt) + omega_e * L_d * i_d + omega_e * lambda_pm
      |
      | where:
      |   omega_e   = P * omega_m         [Electrical angular speed, rad/s]
      |   P         = 4                   [Pole pairs]
      |   L_d, L_q  = 0.35 mH, 0.55 mH    [Direct and quadrature axis inductances]
      |   lambda_pm = 0.0604 Wb           [Permanent magnet flux linkage]
      |
      | 3. FEEDFORWARD DECOUPLING FORMULAS:
      |   Vd_ff = - omega_e * L_q * i_q
      |   Vq_ff = + omega_e * (L_d * i_d + lambda_pm)
      |
      | Voltage commands to inverter:
      |   v_d* = v_d_PI + Vd_ff
      |   v_q* = v_q_PI + Vq_ff
      |
      | 4. WHY IT IS NEEDED:
      | - Nonlinear Decoupling: In IPMSMs, d and q dynamics are strongly coupled through
      |   rotor velocity. Without feedforward, i_q transients disturb i_d and vice versa.
      | - High-Speed Back-EMF & Cross-Coupling Rejection: At maximum speed (20,000 RPM),
      |   omega_e reaches ~8,377 rad/s, producing back-EMF > 500 V and cross-coupling > 200 V.
      |   Without feedforward, the feedback PI integrators must synthesize these huge voltages
      |   purely through tracking error, resulting in severe phase lag, overshoot, and windup.
      | - Ideal Linear SISO Plant: Feedforward cancels the coupling voltages, reducing the
      |   plant seen by the PI controllers to two independent linear first-order SISO loops:
      |     v_d_PI ≈ R_s * i_d + L_d * (di_d/dt)
      |     v_q_PI ≈ R_s * i_q + L_q * (di_q/dt)
      |   ensuring uniform 800 Hz current loop bandwidth across the entire speed envelope.
  speed_rads : Inport
  id : Inport  Port=2
  iq : Inport  Port=3
  FluxPM : Constant  Value=single(pmsm.fl)  OutDataTypeStr=single
  Gain_Ld : Gain  Gain=single(pmsm.Ld)  OutDataTypeStr=single
  Gain_P : Gain  Gain=single(pmsm.P)  OutDataTypeStr=single
  Gain_minus_Lq : Gain  Gain=single(-pmsm.Lq)  OutDataTypeStr=single
  Prod_Vd : Product
  Prod_Vq : Product
  Sum_flux : Sum
  Vd_ff : Outport
  Vq_ff : Outport  Port=2
  wires:
  speed_rads/1 -> Gain_P/1
  Gain_P/1 -> Prod_Vd/2, Prod_Vq/1
  Prod_Vd/1 -> Gain_minus_Lq/1
  Gain_minus_Lq/1 -> Vd_ff/1
  id/1 -> Gain_Ld/1
  Gain_Ld/1 -> Sum_flux/1
  FluxPM/1 -> Sum_flux/2
  Sum_flux/1 -> Prod_Vq/2
  Prod_Vq/1 -> Vq_ff/1
  iq/1 -> Prod_Vd/1

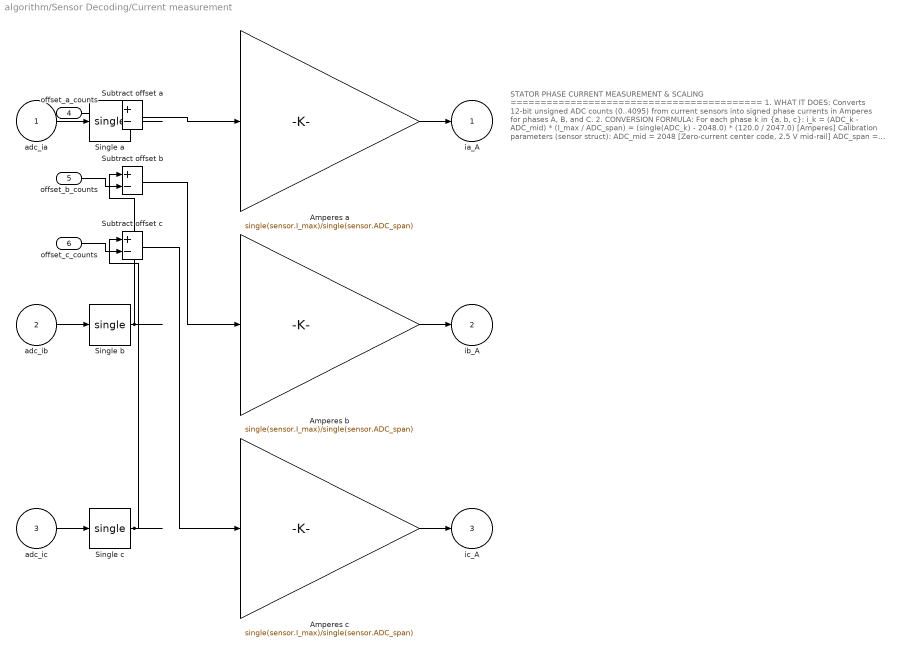
== system algorithm/Sensor Decoding/Current measurement ==
  note: STATOR PHASE CURRENT MEASUREMENT & SCALING
      | ==========================================
      | 1. WHAT IT DOES:
      | Converts 12-bit unsigned ADC counts (0..4095) from current sensors into signed
      | phase currents in Amperes for phases A, B, and C.
      |
      | 2. CONVERSION FORMULA:
      | For each phase k in {a, b, c}:
      |   i_k = (ADC_k - ADC_mid) * (I_max / ADC_span)
      |       = (single(ADC_k) - 2048.0) * (120.0 / 2047.0)  [Amperes]
      |
      | Calibration parameters (sensor struct):
      |   ADC_mid  = 2048   [Zero-current center code, 2.5 V mid-rail]
      |   ADC_span = 2047   [Unipolar count span]
      |   I_max    = 120.0  [Transducer full-scale current, A]
      |
      | 3. WHY IT IS NEEDED:
      | Hall-effect current sensors produce an analog voltage centered at 2.5 V (count 2048)
      | for 0 A, swinging between 0 V (count 0, ≈ -120 A) and 5 V (count 4095, +120 A).
      | This block converts discrete integer ADC codes to physical currents for Clarke transformation.
  adc_ia : Inport  OutDataTypeStr=uint16
  adc_ib : Inport  Port=2  OutDataTypeStr=uint16
  adc_ic : Inport  Port=3  OutDataTypeStr=uint16
  offset_a_counts : Inport  Port=4
  offset_b_counts : Inport  Port=5
  offset_c_counts : Inport  Port=6
  Amperes a : Gain  Gain=single(sensor.I_max)/single(sensor.ADC_span)
  Amperes b : Gain  Gain=single(sensor.I_max)/single(sensor.ADC_span)
  Amperes c : Gain  Gain=single(sensor.I_max)/single(sensor.ADC_span)
  Single a : DataTypeConversion  OutDataTypeStr=single
  Single b : DataTypeConversion  OutDataTypeStr=single
  Single c : DataTypeConversion  OutDataTypeStr=single
  Subtract offset a : Sum  Inputs=+-
  Subtract offset b : Sum  Inputs=+-
  Subtract offset c : Sum  Inputs=+-
  ia_A : Outport
  ib_A : Outport  Port=2
  ic_A : Outport  Port=3
  wires:
  Amperes c/1 -> ic_A/1
  Amperes a/1 -> ia_A/1
  Amperes b/1 -> ib_A/1
  Single b/1 -> Subtract offset b/1
  Single c/1 -> Subtract offset c/1
  adc_ia/1 -> Single a/1
  Single a/1 -> Subtract offset a/1
  adc_ib/1 -> Single b/1
  adc_ic/1 -> Single c/1
  offset_a_counts/1 -> Subtract offset a/2
  Subtract offset a/1 -> Amperes a/1
  offset_b_counts/1 -> Subtract offset b/2
  Subtract offset b/1 -> Amperes b/1
  offset_c_counts/1 -> Subtract offset c/2
  Subtract offset c/1 -> Amperes c/1
